simulink model "LQR_Based_Optimal_Design_Simulink_with_1_State"  (R2021a)
settings: Solver=VariableStepAuto  StartTime=0.0  StopTime=t_final_new  RelTol=1e-3
undefined symbols (not defined in the file): A, B, C, K_new, Ki_new, ref_sig_new
settings Model: Creator=MuhammadQaisarAli  LastModifiedBy=MuhammadQaisarAli

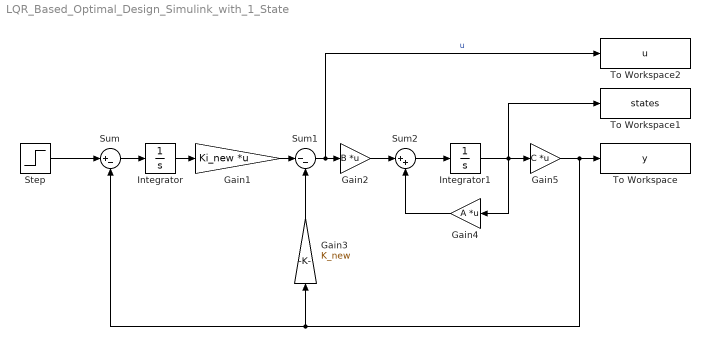
== system LQR_Based_Optimal_Design_Simulink_with_1_State ==
  Gain1 : Gain  Gain=Ki_new  Multiplication=Matrix(K*u)
  Gain2 : Gain  Gain=B  Multiplication=Matrix(K*u)
  Gain3 : Gain  Gain=K_new
  Gain4 : Gain  Gain=A  Multiplication=Matrix(K*u)
  Gain5 : Gain  Gain=C  Multiplication=Matrix(K*u)
  Integrator : Integrator
  Integrator1 : Integrator
  Step : Step  Time=0  After=ref_sig_new  SampleTime=0
  Sum : Sum  Inputs=|+-
  Sum1 : Sum  Inputs=|--
  Sum2 : Sum  Inputs=|++
  To Workspace : ToWorkspace  VariableName=y  SaveFormat=Structure With Time  SampleTime=-1
  To Workspace1 : ToWorkspace  VariableName=states  SaveFormat=Structure With Time  SampleTime=-1
  To Workspace2 : ToWorkspace  VariableName=u  SaveFormat=Structure With Time  SampleTime=-1
  wires:
  Sum/1 -> Integrator/1
  Integrator/1 -> Gain1/1
  Gain1/1 -> Sum1/1
  Sum1/1 -> To Workspace2/1, Gain2/1  "u"
  Gain2/1 -> Sum2/1
  Sum2/1 -> Integrator1/1
  Integrator1/1 -> Gain4/1, To Workspace1/1, Gain5/1
  Gain4/1 -> Sum2/2
  Gain3/1 -> Sum1/2
  Gain5/1 -> Gain3/1, Sum/2, To Workspace/1
  Step/1 -> Sum/1
